simulink model "chap4_3sim"  (Simulink 8.3)
settings: Solver=ode45  StartTime=0.0  StopTime=30  RelTol=1e-3
libraries: fuzblock x1
settings Model: Creator=Prof_Liu  LastModifiedBy=Prof_Liu
settings DataIOCC: SignalLoggingName=sigsOut
settings DebuggingCC: SaveWithParameterizedLinksMsg=none  SignalResolutionControl=TryResolveAllWithWarning  SolverPrmCheckMsg=none  MultiTaskDSMMsg=warning  MultiTaskCondExecSysMsg=none  StateNameClashWarn=none
settings HardwareCC: TargetUnknown=on
settings RTWCC: IncludeERTFirstTime=on

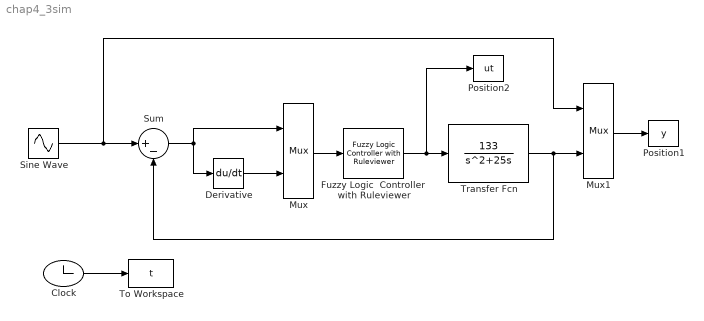
== system chap4_3sim ==
  Clock : Clock
  Derivative : Derivative
  Fuzzy Logic  Controller  with Ruleviewer : fuzblock/Fuzzy Logic  Controller  with Ruleviewer  fismatrix=a2  Ts=2
      link override Fuzzy Logic Controller: fis=a2
  Mux : Mux  Inputs=2
  Mux1 : Mux  Inputs=2
  Position1 : ToWorkspace  VariableName=y  SampleTime=-1
  Position2 : ToWorkspace  VariableName=ut  SampleTime=-1
  Sine Wave : Sin  SampleTime=0
  Sum : Sum  Inputs=|+-  SaturateOnIntegerOverflow=on  InputSameDT=on  OutDataTypeStr=Inherit: Same as first input
  To Workspace : ToWorkspace  VariableName=t  SampleTime=-1
  Transfer Fcn : TransferFcn  Numerator=[133]  Denominator=[1 25 0]
  wires:
  Mux/1 -> Fuzzy Logic  Controller  with Ruleviewer/1
  Derivative/1 -> Mux/2
  Sum/1 -> Mux/1, Derivative/1
  Sine Wave/1 -> Mux1/1, Sum/1
  Mux1/1 -> Position1/1
  Transfer Fcn/1 -> Mux1/2, Sum/2
  Fuzzy Logic  Controller  with Ruleviewer/1 -> Position2/1, Transfer Fcn/1
  Clock/1 -> To Workspace/1
